simulink model "cruise_control_model"  (R2025b)
settings: Solver=VariableStepAuto  StartTime=0.0  StopTime=410  RelTol=1e-2
values from neighbouring files (symbols this model uses):
  Air_Density = 1.225    [Script_Cruise_Control.m]
  auxiliary_load = [0 0 load load 0 0 load load 0 0 load load 0 0 load load 0 0 load load]    [Script_Cruise_Control.m]
  Control_Switch = 0    [Script_Cruise_Control.m]
  Cruise_Speed = 55    [Script_Cruise_Control.m]
  Damping = 0.0018    [Script_Cruise_Control.m]
  Drag_Coefficient = 0.275    [Script_Cruise_Control.m]
  Dynamic_Radius = 0.3346    [Script_Cruise_Control.m]
  Frontal_Area = 2.414    [Script_Cruise_Control.m]
  Gears = 10.65    [Script_Cruise_Control.m]
  Gravity = 9.81    [Script_Cruise_Control.m]
  Inductance = 4.0e-6    (= 4e-06)    [Script_Cruise_Control.m]
  Ke = 0.0125    [Script_Cruise_Control.m]
  Kt = 0.30    (= 0.3)    [Script_Cruise_Control.m]
  longitudinal_distance = [0.00	16.67	33.33	50.00	66.67	83.33	100.00	116.67	133.33	150.00	166.67	183.33	200.00	216.67	233.33	250.00	266.67	283.33	300.00	316.67	333.33	350.00	366.67	383.33	400.00	416.67	433.33	450.00	466.67	483.33	500.00	516.67	533.33	550.00	566.67	583.33	600.00	616.67	633.33	650.00	666.67	683.33	700.00	716.67	733.33	750.00	766.67	783.33	800.00	816.67	833.33	850.00	866.67	883.33	900.00	916.67	933.33	950.00	 ...(+4343 chars)    [Script_Cruise_Control.m]
  Resistance = 0.0200    (= 0.02)    [Script_Cruise_Control.m]
  road_elevation = [0.00	0.63	0.70	1.05	0.36	2.05	2.11	3.91	4.17	5.05	3.60	2.90	4.14	3.50	4.08	3.72	3.59	2.24	0.97	1.95	1.91	1.11	0.34	1.20	1.15	1.66	2.06	2.81	3.21	1.87	2.25	3.37	4.10	1.72	1.45	1.13	1.45	0.93	0.93	2.54	3.39	3.65	2.73	2.66	2.81	2.25	1.92	2.33	3.89	1.44	0.35	1.47	2.05	1.78	2.19	1.21	0.19	0.51	2.03	2.78	2.27	3.15	2.91	2.18	1.73	1.12	0.91	1.47	0.41	0.76	1.90	2.05	2.75	2.70	4.71	5.64	3.82	3.86	2.05	3.08 ...(+2942 chars)    [Script_Cruise_Control.m]
  Rolling_Resistance_Factor = 0.011    [Script_Cruise_Control.m]
  time = [0 100 101 233 234 404 405 465 466 512 513 580 585 600 605 750 755 805 810 1000]    [Script_Cruise_Control.m]
  Total_Mass = Driver_Mass + Vehicle_Mass    (= 1720)    [Script_Cruise_Control.m]
  wind_speed = [0.00	0.00	0.00	0.00	0.00	0.00	0.00	32.95	5.35	3.83	0.00	0.00	0.31	9.19	8.02	0.00	5.44	0.00	0.00	17.24	22.27	0.00	0.00	0.00	0.19	1.54	26.13	9.62	22.24	0.00	4.79	14.01	30.38	0.00	5.01	0.00	3.05	0.00	5.02	37.09	13.32	14.98	0.00	0.00	0.00	3.11	10.57	0.00	18.54	0.00	0.00	15.44	33.60	14.78	2.99	0.00	0.00	19.29	34.28	15.58	0.00	6.49	0.00	5.68	3.62	14.26	9.57	0.00	0.00	13.54	35.14	27.56	8.15	0.00	27.31	4 ...(+2787 chars)    [Script_Cruise_Control.m]
libraries: slpidlib x1
settings Model: Creator=M Wasib  LastModifiedBy=M Wasib
settings DebuggingCC: AlgebraicLoopMsg=none

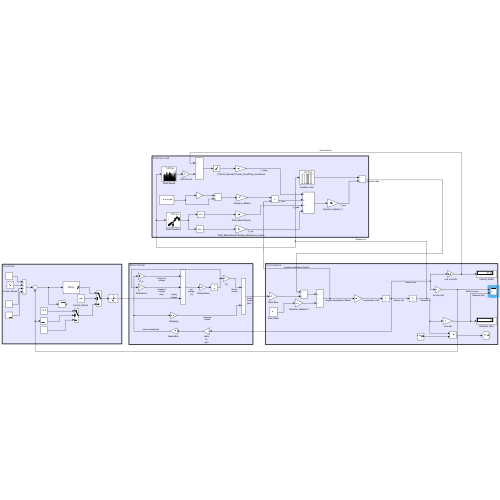
[thumbnail: Simulink's stored preview of the top-level diagram]
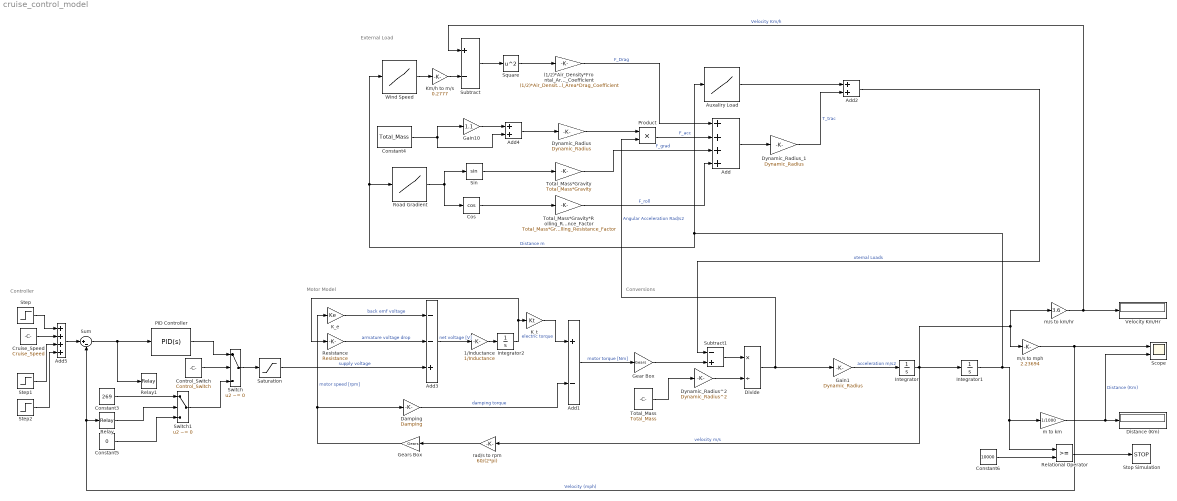
== system cruise_control_model ==
  note: Conversions
  note: External Load
  note: Controller
  note: Motor Model
  (1/2)*Air_Density*Frontal_Area*Drag_Coefficient : Gain  Gain=(1/2)*Air_Density*Frontal_Area*Drag_Coefficient
  1/Inductance : Gain  Gain=1/Inductance
  Add : Sum  Inputs=++++
  Add1 : Sum  Inputs=+-
  Add2 : Sum
  Add3 : Sum  Inputs=--+
  Add4 : Sum
  Add5 : Sum  Inputs=++++
  Auxaliry Load : Lookup_n-D  NumberOfTableDimensions=1  BreakpointsForDimension1=time  Table=auxiliary_load  InternalRulePriority=Speed  RndMeth=Simplest
  Constant3 : Constant  Value=269
  Constant4 : Constant  Value=Total_Mass
  Constant5 : Constant  Value=0
  Constant6 : Constant  Value=10000
  "Control_Switch " : Constant  Value=Control_Switch
  Cos : Trigonometry  Operator=cos
  Cruise_Speed : Constant  Value=Cruise_Speed
  Damping : Gain  Gain=Damping
  Distance (Km) : Display
  Divide : Product  Inputs=*/
  Dynamic_Radius : Gain  Gain=Dynamic_Radius
  Dynamic_Radius^2 : Gain  Gain=Dynamic_Radius^2
  Dynamic_Radius_1 : Gain  Gain=Dynamic_Radius
  Gain1 : Gain  Gain=Dynamic_Radius
  Gain10 : Gain  Gain=1.1
  Gear Box : Gain  Gain=Gears
  Gears Box : Gain  Gain=Gears
  Integrator : Integrator
  Integrator1 : Integrator
  Integrator2 : Integrator
  K_e : Gain  Gain=Ke
  K_t : Gain  Gain=Kt
  Km/h to m/s : Gain  Gain=0.2777
  PID Controller : slpidlib/PID Controller  Controller=PID  Form=Parallel  TimeDomain=Continuous-time  UseExternalTs=off  SampleTime=-1  IntegratorMethod=Forward Euler  FilterMethod=Forward Euler  ControllerParametersSource=internal  P=36.89883949  I=23.3695050  UseKiTs=off  D=0.1596060  UseExternalDerivativeSource=off  N=23.85  UseFilter=on  TunerSelectOption=Transfer Function Based (PID Tuner App)  InitialConditionSource=internal  InitialConditionForIntegrator=0  InitialConditionForFilter=0  DifferentiatorICPrevScaledInput=0  ExternalReset=none  TrackingMode=off  Kt=1  LimitOutput=on  SatLimitsSource=internal  UpperSaturationLimit=350  LowerSaturationLimit=0  LinearizeAsGain=off  AntiWindupMode=none  Kb=1  LimitIntegrator=off  UpperIntegratorSaturationLimit=inf  LowerIntegratorSaturationLimit=-inf  POutMin=[]  POutMax=[]  IOutMin=[]  IOutMax=[]  DOutMin=[]  DOutMax=[]  NOutMin=[]  NOutMax=[]  SumOutMin=[]  SumOutMax=[]  SaturationOutMin=[]  SaturationOutMax=[]  PParamMin=[]  PParamMax=[]  IParamMin=[]  IParamMax=[]  DParamMin=[]  DParamMax=[]  NParamMin=[]  NParamMax=[]  KbParamMin=[]  KbParamMax=[]  KtParamMin=[]  KtParamMax=[]  KbOutMin=[]  KbOutMax=[]  KtOutMin=[]  KtOutMax=[]  IntegratorOutMin=[]  IntegratorOutMax=[]  FilterOutMin=[]  FilterOutMax=[]  SumI1OutMin=[]  SumI1OutMax=[]  SumI2OutMin=[]  SumI2OutMax=[]  SumI3OutMin=[]  SumI3OutMax=[]  SumI4OutMin=[]  SumI4OutMax=[]  SumDOutMin=[]  SumDOutMax=[]  DifferentiatorOutMin=[]  DifferentiatorOutMax=[]  FilterDiffOutCoefMin=[]  FilterDiffOutCoefMax=[]  ReciprocalOutMin=[]  ReciprocalOutMax=[]  SumDenOutMin=[]  SumDenOutMax=[]  SumNumOutMin=[]  SumNumOutMax=[]  DivideOutMin=[]  DivideOutMax=[]  UdiffTsProdOutMin=[]  UdiffTsProdOutMax=[]  NTsProdOutMin=[]  NTsProdOutMax=[]  UintegralTsProdOutMin=[]  UintegralTsProdOutMax=[]  UngainTsProdOutMin=[]  UngainTsProdOutMax=[]  ClampingZeroOutDataTypeStr=Inherit: Inherit via back propagation  ClampingZeroOutMin=[]  ClampingZeroOutMax=[]  FilterDenConstantOutDataTypeStr=Inherit: Inherit via back propagation  FilterDenConstantOutMin=[]  FilterDenConstantOutMax=[]  PCopyOutDataTypeStr=Inherit: Inherit via back propagation  PCopyOutMin=[]  PCopyOutMax=[]  NCopyOutDataTypeStr=Inherit: Inherit via back propagation  NCopyOutMin=[]  NCopyOutMax=[]  IntegratorContinuousStateAttributes=''  IntegratorStateMustResolveToSignalObject=off  IntegratorRTWStateStorageClass=Auto  FilterContinuousStateAttributes=''  FilterStateMustResolveToSignalObject=off  FilterRTWStateStorageClass=Auto  ParallelPVariant=InternalParameters  IdealPVariant=Disabled  IVariant=InternalParameters  DVariant=InternalParameters  IntegratorVariant=Continuous  SatVariant=Enabled  AWVariant=Passthrough  PCopyVariant=Disabled  TRVariant=Disabled  FdbkBlocksVariant=Forward  IdealPFdbkVariant=Disabled  SatFdbkVariant=Disabled  DerivativeFilterVariant=ContFilter  NVariant=InternalParameters  NCopyVariant=Disabled  FilterICVariant=InternalICsFilter  IntegratorICVariant=InternalICs  ExternalResetVariant=Disabled  TRSumVariant=Passthrough  SumFdbkVariant=Disabled  SumVariant=Sum_PID  TsampFilterVariant=InternalTs  TsampNgainVariant=Passthrough  TsampIntegralVariant=Disabled_SignalSpec  ExternalSaturationOutDataTypeStr=Inherit: Same as second input  DerivativeSourceVariant=ErrorSignal  PreIntVariant=InternalPreInt
  Product : Product
  Relational Operator : RelationalOperator  OutDataTypeStr=boolean  RndMeth=Simplest  InputSameDT=off
  Relay : Relay  OnSwitchValue=55.5  OffSwitchValue=54.5  OnOutputValue=0  OffOutputValue=1
  Relay1 : Relay  OnSwitchValue=0.5  OffSwitchValue=-0.5  OnOutputValue=269
  Resistance : Gain  Gain=Resistance
  Road Gradient : Lookup_n-D  NumberOfTableDimensions=1  BreakpointsForDimension1=longitudinal_distance  Table=road_elevation  InternalRulePriority=Speed  RndMeth=Simplest
  Saturation : Saturate  UpperLimit=269  LowerLimit=0
  Scope : Scope  NumInputPorts=2
      settings: ActiveDisplayYMinimum=-6.9387508698755047  ActiveDisplayYMaximum=62.448757753373634
  Sin : Trigonometry
  Square : Math  Operator=square
  Step : Step  Time=80  After=10  SampleTime=0
  Step1 : Step  Time=160  After=15  SampleTime=0
  Step2 : Step  Time=260  After=-30  SampleTime=0
  Stop Simulation : Stop
  Subtract : Sum  Inputs=+-
  Subtract1 : Sum  Inputs=-+
  Sum : Sum  Inputs=|+-
  Switch : Switch  Criteria=u2 ~= 0  SaturateOnIntegerOverflow=off  InputSameDT=off
  Switch1 : Switch  Criteria=u2 ~= 0  SaturateOnIntegerOverflow=off  InputSameDT=off
  Total_Mass : Constant  Value=Total_Mass
  Total_Mass*Gravity : Gain  Gain=Total_Mass*Gravity
  Total_Mass*Gravity*Rolling_Resistance_Factor : Gain  Gain=Total_Mass*Gravity*Rolling_Resistance_Factor
  Velocity Km/Hr : Display
  Wind Speed : Lookup_n-D  NumberOfTableDimensions=1  BreakpointsForDimension1=longitudinal_distance  Table=wind_speed  InternalRulePriority=Speed  RndMeth=Simplest
  m to km : Gain  Gain=1/1000
  m/s to km/hr : Gain  Gain=3.6
  m/s to mph : Gain  Gain=2.23694
  rad/s to rpm : Gain  Gain=60/(2*pi)
  wires:
  Divide/1 -> Gain1/1, Product/2  "Angular Acceleration Rad/s2"
  Constant4/1 -> Gain10/1, Add4/2
  Gain10/1 -> Add4/1
  K_t/1 -> Add1/1  "electric torque"
  Subtract/1 -> Square/1
  Cos/1 -> Total_Mass*Gravity*Rolling_Resistance_Factor/1
  Add1/1 -> Gear Box/1  "motor torque [Nm]"
  Integrator/1 -> rad/s to rpm/1, Integrator1/1, m/s to mph/1, m/s to km/hr/1  "velocity m/s"
  rad/s to rpm/1 -> Gears Box/1
  Total_Mass*Gravity/1 -> Add/3  "F_grad"
  Dynamic_Radius/1 -> Product/1
  Dynamic_Radius^2/1 -> Divide/2
  Constant6/1 -> Relational Operator/2
  m to km/1 -> Scope/2, Distance (Km)/1  "Distance (Km)"
  Integrator1/1 -> m to km/1, Relational Operator/1, Wind Speed/1, Road Gradient/1, Auxaliry Load/1  "Distance m"
  Gear Box/1 -> Subtract1/2
  K_e/1 -> Add3/1  "back emf voltage"
  Total_Mass/1 -> Dynamic_Radius^2/1
  Constant5/1 -> Switch1/3
  Road Gradient/1 -> Sin/1, Cos/1
  Auxaliry Load/1 -> Add2/1
  1/Inductance/1 -> Integrator2/1
  Gears Box/1 -> Damping/1, K_e/1  "motor speed [rpm]"
  Switch/1 -> Saturation/1
  Total_Mass*Gravity*Rolling_Resistance_Factor/1 -> Add/4  "F_roll"
  PID Controller/1 -> Switch/1
  Saturation/1 -> Add3/3  "supply voltage"
  Subtract1/1 -> Divide/1
  Integrator2/1 -> Resistance/1, K_t/1
  Sin/1 -> Total_Mass*Gravity/1
  m/s to km/hr/1 -> Subtract/1, Velocity Km/Hr/1  "Velocity Km/h"
  Gain1/1 -> Integrator/1  "acceleration m/s2"
  Add3/1 -> 1/Inductance/1  "net voltage [V]"
  Constant3/1 -> Switch1/1
  Product/1 -> Add/2  "F_acc"
  Add4/1 -> Dynamic_Radius/1
  Relay/1 -> Switch1/2
  m/s to mph/1 -> Relay/1, Sum/2, Scope/1  "Velocity (mph)"
  "Control_Switch "/1 -> Switch/2
  Damping/1 -> Add1/2  "damping torque"
  (1/2)*Air_Density*Frontal_Area*Drag_Coefficient/1 -> Add/1  "F_Drag"
  Square/1 -> (1/2)*Air_Density*Frontal_Area*Drag_Coefficient/1
  Resistance/1 -> Add3/2  "armature voltage drop"
  Relational Operator/1 -> Stop Simulation/1
  Add2/1 -> Subtract1/1  "xternal Loads"
  Wind Speed/1 -> Km/h to m/s/1
  Km/h to m/s/1 -> Subtract/2
  Add/1 -> Dynamic_Radius_1/1
  Dynamic_Radius_1/1 -> Add2/2  "T_trac"
  Sum/1 -> Relay1/1, PID Controller/1
  Cruise_Speed/1 -> Add5/2
  Add5/1 -> Sum/1
  Step/1 -> Add5/1
  Step1/1 -> Add5/3
  Step2/1 -> Add5/4
  Switch1/1 -> Switch/3
